simulink model "SWC_DID_type"  (R2021b)
settings: Solver=FixedStepDiscrete  StartTime=0.0  StopTime=10.0  RelTol=1e-3
(part 1 of 2)
settings Model: DataDictionary=APPTypes.sldd  Creator=FVT23033  LastModifiedBy=FVT23033
settings DataIOCC: SaveFormat=StructureWithTime
settings OptimizationCC: DefaultParameterBehavior=Inlined  EnhancedBackFolding=on  PassReuseOutputArgsAs=Individual arguments  ZeroExternalMemoryAtStartup=off  ZeroInternalMemoryAtStartup=off  OptimizeBlockOrder=speed  DifferentSizesBufferReuse=on  OptimizationCustomize=off  EfficientTunableParamExpr=on
settings DebuggingCC: ParameterTunabilityLossMsg=error
settings HardwareCC: ProdBitPerPointer=32  ProdBitPerSizeT=32  ProdBitPerPtrDiffT=32  ProdLargestAtomicInteger=Long  ProdLargestAtomicFloat=Double  ProdWordSize=32  ProdLongLongMode=on  ProdHWDeviceType=ARM Compatible->ARM Cortex-M
settings SFSimCC: MATLABDynamicMemAlloc=off
settings RTWCC: Description=AUTOSAR  SystemTargetFile=autosar.tlc  GenCodeOnly=on  TemplateMakefile=ert_default_tmf  PortableWordSizes=on
settings CodeAppCC: ForceParamTrailComments=on  IgnoreCustomStorageClasses=off  OperatorAnnotations=on  SimulinkDataObjDesc=on  SFDataObjDesc=on  InsertBlockDesc=on
settings STFCustomTargetCC: TargetLangStandard=C99 (ISO)  UtilityFuncGeneration=Shared location  MultiwordLength=256  ParMdlRefBuildCompliant=on  CompOptLevelCompliant=on  IncludeMdlTerminateFcn=off  CombineOutputUpdateFcns=on  SuppressErrorStatus=on  ERTCustomFileBanners=on  SupportNonFinite=off  SupportComplex=off  SupportContinuousTime=off  SupportNonInlinedSFcns=off  RemoveResetFunc=on  MATLABClassNameForMDSCustomization=Simulink.SoftwareTarget.ERTCustomization  AutosarCompliant=on  GRTInterface=off  UseToolchainInfoCompliant=on  GenerateSharedConstants=off  LookupTableObjectStructAxisOrder=2,1,3,4,...  LUTObjectStructOrderEvenSpacing=Size,Table,Breakpoints  SystemTargetFile=autosar.tlc
settings ERTTargetCC: TargetLangStandard=C99 (ISO)  UtilityFuncGeneration=Shared location  ConcurrentExecutionCompliant=off  IncludeMdlTerminateFcn=off  SuppressErrorStatus=on  SupportNonFinite=off  SupportComplex=off  ModelStepFunctionPrototypeControlCompliant=off  CPPClassGenCompliant=off  AutosarCompliant=on  GenerateSharedConstants=off  LookupTableObjectStructAxisOrder=2,1,3,4,...  LUTObjectStructOrderEvenSpacing=Size,Table,Breakpoints  GenerateASAP2=on  InlinedParameterPlacement=NonHierarchical  ERTCustomFileTemplate=example_file_process.tlc  ConvertIfToSwitch=off  SuppressUnreachableDefaultCases=off  BooleanTrueId=true_MatlabRTW  BooleanFalseId=false_MatlabRTW

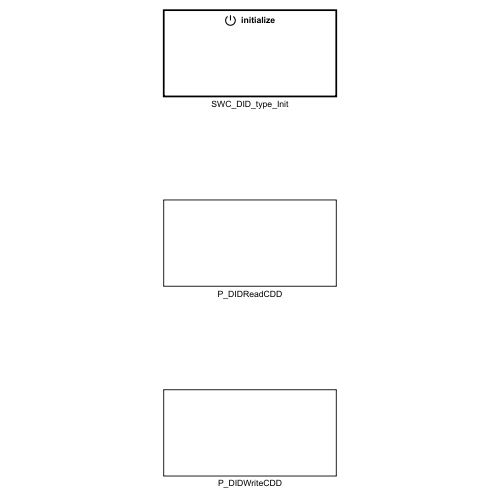
[thumbnail: Simulink's stored preview of the top-level diagram]
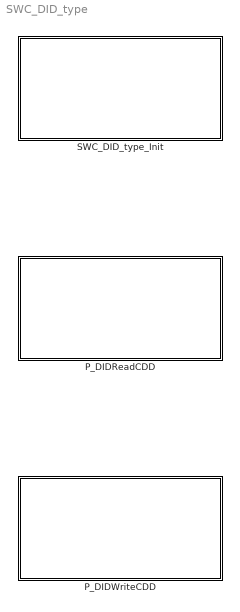
== system SWC_DID_type ==
  P_DIDReadCDD : Subsystem
  P_DIDWriteCDD : Subsystem
  SWC_DID_type_Init : Subsystem

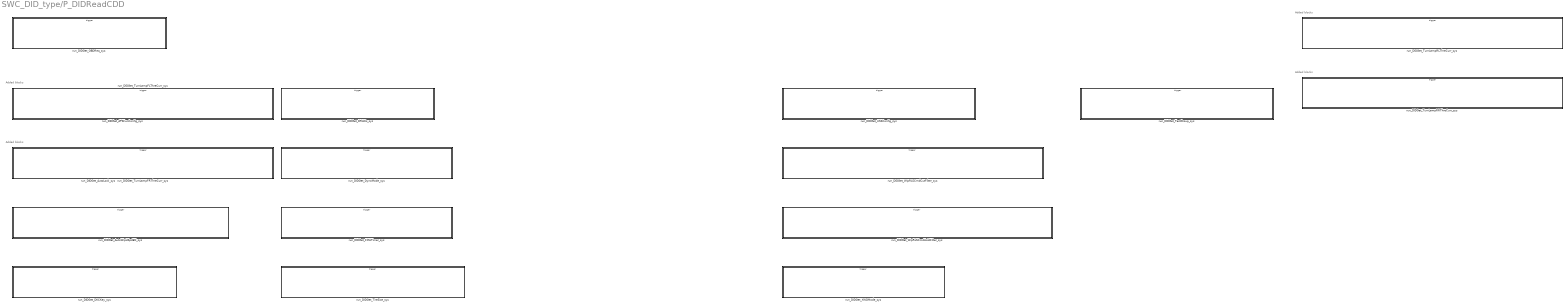
== system SWC_DID_type/P_DIDReadCDD ==
  note: Added blocks
  note: Added blocks
  note: Added blocks
  note: Added blocks
  run_DIDGet_APSFunConfig_sys : Subsystem
  run_DIDGet_AutoLock_sys : Subsystem
  run_DIDGet_AutoWipHSpdEN_sys : Subsystem
  run_DIDGet_DKCKey_sys : Subsystem
  run_DIDGet_DRLDis_sys : Subsystem
  run_DIDGet_DynoMode_sys : Subsystem
  run_DIDGet_FMHTimer_sys : Subsystem
  run_DIDGet_OBDReq_sys : Subsystem
  run_DIDGet_TestGroup_sys : Subsystem
  run_DIDGet_TireSize_sys : Subsystem
  run_DIDGet_TurnLampFLThreCurr_sys : Subsystem
  run_DIDGet_TurnLampFRThreCurr_sys : Subsystem
  run_DIDGet_TurnLampRLThreCurr_sys : Subsystem
  run_DIDGet_TurnLampRRThreCurr_sys : Subsystem
  run_DIDGet_USSConfig_sys : Subsystem
  run_DIDGet_WipRLSCmdCutFilter_sys : Subsystem
  run_DIDGet_WipRLSCmdHoldFilter_sys : Subsystem
  run_DIDGet_XWDMode_sys : Subsystem

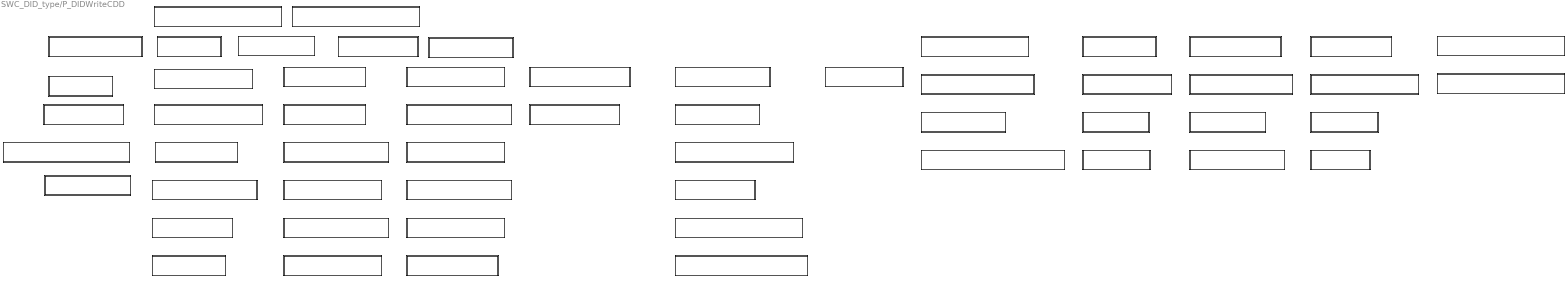
== system SWC_DID_type/P_DIDWriteCDD ==
  note: Added blocks
  note: Added blocks
  note: Added blocks
  note: Added blocks
  run_DIDSet_APPD_sys : Subsystem
  run_DIDSet_APPE_sys : Subsystem
  run_DIDSet_APPPedalZP_sys : Subsystem
  run_DIDSet_APSFunConfig_sys : Subsystem
  run_DIDSet_AutoLock_sys : Subsystem
  run_DIDSet_AutoWipHSpdEN_sys : Subsystem
  run_DIDSet_CALID_sys : Subsystem
  run_DIDSet_CDEODT_sys : Subsystem
  run_DIDSet_CLRDIST_sys : Subsystem
  run_DIDSet_DKCBLESta_sys : Subsystem
  run_DIDSet_DKCKey_sys : Subsystem
  run_DIDSet_DKCSta_sys : Subsystem
  run_DIDSet_DRLDis_sys : Subsystem
  run_DIDSet_DoorNFCAnchorSta_sys : Subsystem
  run_DIDSet_DynoMode_sys : Subsystem
  run_DIDSet_ECUNAME_sys : Subsystem
  run_DIDSet_FDDKCCoordXY_sys : Subsystem
  run_DIDSet_FMHTimer_sys : Subsystem
  run_DIDSet_LFLowPresThre_sys : Subsystem
  run_DIDSet_LFSensorID_sys : Subsystem
  run_DIDSet_LIDAAnchorSta_sys : Subsystem
  run_DIDSet_LRLowPresThre_sys : Subsystem
  run_DIDSet_LRSensorID_sys : Subsystem
  run_DIDSet_MILDIST_sys : Subsystem
  run_DIDSet_NUMPSATRIPSFLTMEMCLR_sys : Subsystem
  run_DIDSet_NVMPedalZP_sys : Subsystem
  run_DIDSet_OBDReq_sys : Subsystem
  run_DIDSet_ODOMETER_sys : Subsystem
  run_DIDSet_PKE_sys : Subsystem
  run_DIDSet_PSA_sys : Subsystem
  run_DIDSet_ProtocolId_sys : Subsystem
  run_DIDSet_QTYPSATRIPS_sys : Subsystem
  run_DIDSet_RFLowPresThre_sys : Subsystem
  run_DIDSet_RFSensorID_sys : Subsystem
  run_DIDSet_RRLowPresThre_sys : Subsystem
  run_DIDSet_RRSensorID_sys : Subsystem
  run_DIDSet_RUNTM_sys : Subsystem
  run_DIDSet_SensorMode_sys : Subsystem
  run_DIDSet_TPMSLearnSta_sys : Subsystem
  run_DIDSet_TestGroup_sys : Subsystem
  run_DIDSet_TireSize_sys : Subsystem
  run_DIDSet_TurnLampFLThreCurr_sys : Subsystem
  run_DIDSet_TurnLampFRThreCurr_sys : Subsystem
  run_DIDSet_TurnLampRLThreCurr_sys : Subsystem
  run_DIDSet_TurnLampRRThreCurr_sys : Subsystem
  run_DIDSet_UIDSta_sys : Subsystem
  run_DIDSet_USSConfig_sys : Subsystem
  run_DIDSet_UWBAnchorSta_sys : Subsystem
  run_DIDSet_VIN_sys : Subsystem
  run_DIDSet_VSS_sys : Subsystem
  run_DIDSet_WhlPres_sys : Subsystem
  run_DIDSet_WhlSensorBattSta_sys : Subsystem
  run_DIDSet_WhlTmp_sys : Subsystem
  run_DIDSet_WipRLSCmdCutFilter_sys : Subsystem
  run_DIDSet_WipRLSCmdHoldFilter_sys : Subsystem
  run_DIDSet_XWDMode_sys : Subsystem

== system SWC_DID_type/SWC_DID_type_Init ==
  Event Listener : EventListener  EventName=reset

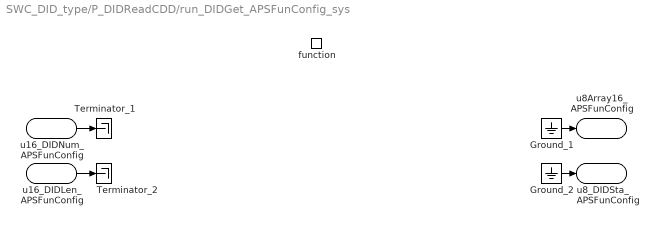
== system SWC_DID_type/P_DIDReadCDD/run_DIDGet_APSFunConfig_sys ==
  function : TriggerPort  TriggerType=function-call  IsSimulinkFunction=on  FunctionName=run_DIDGet_APSFunConfig  VariantControl=(inherit)
  Ground_1 : Ground
  Ground_2 : Ground
  Terminator_1 : Terminator
  Terminator_2 : Terminator
  u16_DIDNum_APSFunConfig : ArgIn  OutDataTypeStr=uint16  ArgumentName=u16_DIDNum_APSFunConfig
  u16_DIDLen_APSFunConfig : ArgIn  Port=2  OutDataTypeStr=uint16  ArgumentName=u16_DIDLen_APSFunConfig
  u8Array16_APSFunConfig : ArgOut  OutDataTypeStr=uint8  PortDimensions=16  ArgumentName=u8Array16_APSFunConfig
  u8_DIDSta_APSFunConfig : ArgOut  Port=2  OutDataTypeStr=uint8  ArgumentName=u8_DIDSta_APSFunConfig
  wires:
  u16_DIDNum_APSFunConfig/1 -> Terminator_1/1
  u16_DIDLen_APSFunConfig/1 -> Terminator_2/1
  Ground_1/1 -> u8Array16_APSFunConfig/1
  Ground_2/1 -> u8_DIDSta_APSFunConfig/1

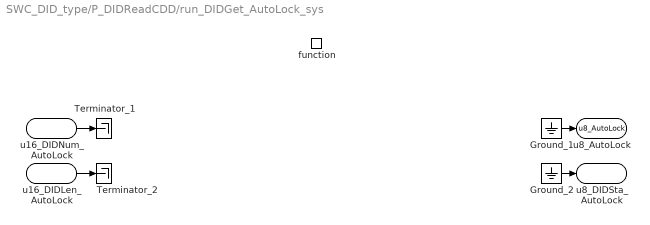
== system SWC_DID_type/P_DIDReadCDD/run_DIDGet_AutoLock_sys ==
  function : TriggerPort  TriggerType=function-call  IsSimulinkFunction=on  FunctionName=run_DIDGet_AutoLock  VariantControl=(inherit)
  Ground_1 : Ground
  Ground_2 : Ground
  Terminator_1 : Terminator
  Terminator_2 : Terminator
  u16_DIDNum_AutoLock : ArgIn  OutDataTypeStr=uint16  ArgumentName=u16_DIDNum_AutoLock
  u16_DIDLen_AutoLock : ArgIn  Port=2  OutDataTypeStr=uint16  ArgumentName=u16_DIDLen_AutoLock
  u8_AutoLock : ArgOut  OutDataTypeStr=uint8  ArgumentName=u8_AutoLock
  u8_DIDSta_AutoLock : ArgOut  Port=2  OutDataTypeStr=uint8  ArgumentName=u8_DIDSta_AutoLock
  wires:
  u16_DIDNum_AutoLock/1 -> Terminator_1/1
  u16_DIDLen_AutoLock/1 -> Terminator_2/1
  Ground_1/1 -> u8_AutoLock/1
  Ground_2/1 -> u8_DIDSta_AutoLock/1

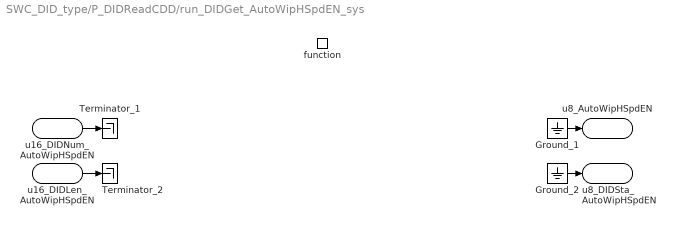
== system SWC_DID_type/P_DIDReadCDD/run_DIDGet_AutoWipHSpdEN_sys ==
  function : TriggerPort  TriggerType=function-call  IsSimulinkFunction=on  FunctionName=run_DIDGet_AutoWipHSpdEN  VariantControl=(inherit)
  Ground_1 : Ground
  Ground_2 : Ground
  Terminator_1 : Terminator
  Terminator_2 : Terminator
  u16_DIDNum_AutoWipHSpdEN : ArgIn  OutDataTypeStr=uint16  ArgumentName=u16_DIDNum_AutoWipHSpdEN
  u16_DIDLen_AutoWipHSpdEN : ArgIn  Port=2  OutDataTypeStr=uint16  ArgumentName=u16_DIDLen_AutoWipHSpdEN
  u8_AutoWipHSpdEN : ArgOut  OutDataTypeStr=uint8  ArgumentName=u8_AutoWipHSpdEN
  u8_DIDSta_AutoWipHSpdEN : ArgOut  Port=2  OutDataTypeStr=uint8  ArgumentName=u8_DIDSta_AutoWipHSpdEN
  wires:
  u16_DIDNum_AutoWipHSpdEN/1 -> Terminator_1/1
  u16_DIDLen_AutoWipHSpdEN/1 -> Terminator_2/1
  Ground_1/1 -> u8_AutoWipHSpdEN/1
  Ground_2/1 -> u8_DIDSta_AutoWipHSpdEN/1

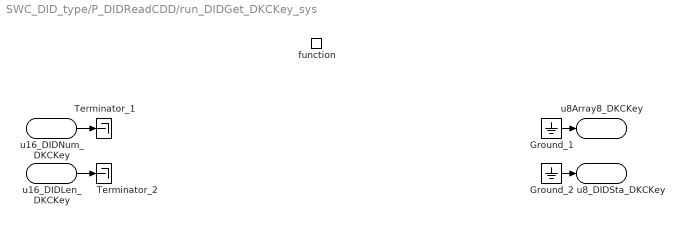
== system SWC_DID_type/P_DIDReadCDD/run_DIDGet_DKCKey_sys ==
  function : TriggerPort  TriggerType=function-call  IsSimulinkFunction=on  FunctionName=run_DIDGet_DKCKey  VariantControl=(inherit)
  Ground_1 : Ground
  Ground_2 : Ground
  Terminator_1 : Terminator
  Terminator_2 : Terminator
  u16_DIDNum_DKCKey : ArgIn  OutDataTypeStr=uint16  ArgumentName=u16_DIDNum_DKCKey
  u16_DIDLen_DKCKey : ArgIn  Port=2  OutDataTypeStr=uint16  ArgumentName=u16_DIDLen_DKCKey
  u8Array8_DKCKey : ArgOut  OutDataTypeStr=uint8  PortDimensions=8  ArgumentName=u8Array8_DKCKey
  u8_DIDSta_DKCKey : ArgOut  Port=2  OutDataTypeStr=uint8  ArgumentName=u8_DIDSta_DKCKey
  wires:
  u16_DIDNum_DKCKey/1 -> Terminator_1/1
  u16_DIDLen_DKCKey/1 -> Terminator_2/1
  Ground_1/1 -> u8Array8_DKCKey/1
  Ground_2/1 -> u8_DIDSta_DKCKey/1

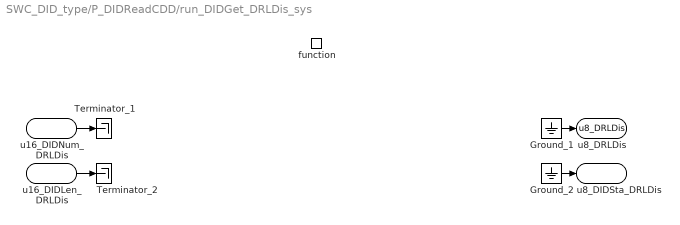
== system SWC_DID_type/P_DIDReadCDD/run_DIDGet_DRLDis_sys ==
  function : TriggerPort  TriggerType=function-call  IsSimulinkFunction=on  FunctionName=run_DIDGet_DRLDis  VariantControl=(inherit)
  Ground_1 : Ground
  Ground_2 : Ground
  Terminator_1 : Terminator
  Terminator_2 : Terminator
  u16_DIDNum_DRLDis : ArgIn  OutDataTypeStr=uint16  ArgumentName=u16_DIDNum_DRLDis
  u16_DIDLen_DRLDis : ArgIn  Port=2  OutDataTypeStr=uint16  ArgumentName=u16_DIDLen_DRLDis
  u8_DRLDis : ArgOut  OutDataTypeStr=uint8  ArgumentName=u8_DRLDis
  u8_DIDSta_DRLDis : ArgOut  Port=2  OutDataTypeStr=uint8  ArgumentName=u8_DIDSta_DRLDis
  wires:
  u16_DIDNum_DRLDis/1 -> Terminator_1/1
  u16_DIDLen_DRLDis/1 -> Terminator_2/1
  Ground_1/1 -> u8_DRLDis/1
  Ground_2/1 -> u8_DIDSta_DRLDis/1

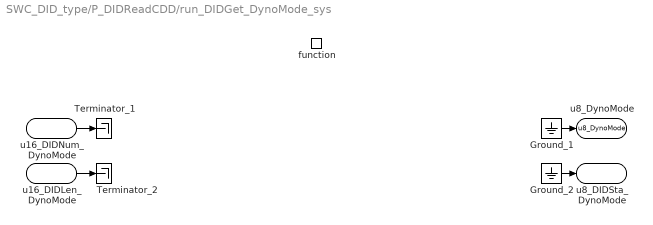
== system SWC_DID_type/P_DIDReadCDD/run_DIDGet_DynoMode_sys ==
  function : TriggerPort  TriggerType=function-call  IsSimulinkFunction=on  FunctionName=run_DIDGet_DynoMode  VariantControl=(inherit)
  Ground_1 : Ground
  Ground_2 : Ground
  Terminator_1 : Terminator
  Terminator_2 : Terminator
  u16_DIDNum_DynoMode : ArgIn  OutDataTypeStr=uint16  ArgumentName=u16_DIDNum_DynoMode
  u16_DIDLen_DynoMode : ArgIn  Port=2  OutDataTypeStr=uint16  ArgumentName=u16_DIDLen_DynoMode
  u8_DynoMode : ArgOut  OutDataTypeStr=uint8  ArgumentName=u8_DynoMode
  u8_DIDSta_DynoMode : ArgOut  Port=2  OutDataTypeStr=uint8  ArgumentName=u8_DIDSta_DynoMode
  wires:
  u16_DIDNum_DynoMode/1 -> Terminator_1/1
  u16_DIDLen_DynoMode/1 -> Terminator_2/1
  Ground_1/1 -> u8_DynoMode/1
  Ground_2/1 -> u8_DIDSta_DynoMode/1

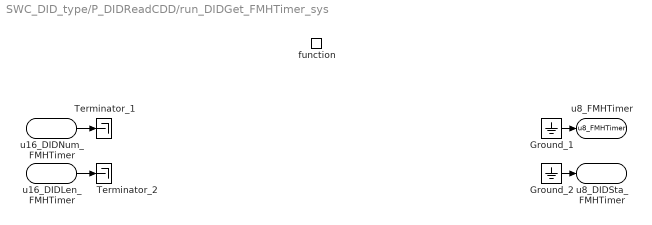
== system SWC_DID_type/P_DIDReadCDD/run_DIDGet_FMHTimer_sys ==
  function : TriggerPort  TriggerType=function-call  IsSimulinkFunction=on  FunctionName=run_DIDGet_FMHTimer  VariantControl=(inherit)
  Ground_1 : Ground
  Ground_2 : Ground
  Terminator_1 : Terminator
  Terminator_2 : Terminator
  u16_DIDNum_FMHTimer : ArgIn  OutDataTypeStr=uint16  ArgumentName=u16_DIDNum_FMHTimer
  u16_DIDLen_FMHTimer : ArgIn  Port=2  OutDataTypeStr=uint16  ArgumentName=u16_DIDLen_FMHTimer
  u8_FMHTimer : ArgOut  OutDataTypeStr=uint8  ArgumentName=u8_FMHTimer
  u8_DIDSta_FMHTimer : ArgOut  Port=2  OutDataTypeStr=uint8  ArgumentName=u8_DIDSta_FMHTimer
  wires:
  u16_DIDNum_FMHTimer/1 -> Terminator_1/1
  u16_DIDLen_FMHTimer/1 -> Terminator_2/1
  Ground_1/1 -> u8_FMHTimer/1
  Ground_2/1 -> u8_DIDSta_FMHTimer/1

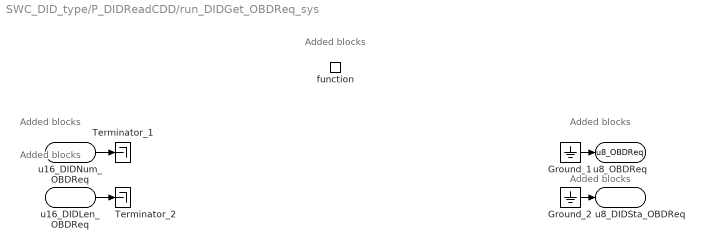
== system SWC_DID_type/P_DIDReadCDD/run_DIDGet_OBDReq_sys ==
  note: Added blocks
  note: Added blocks
  note: Added blocks
  note: Added blocks
  note: Added blocks
  function : TriggerPort  TriggerType=function-call  IsSimulinkFunction=on  FunctionName=run_DIDGet_OBDReq  VariantControl=(inherit)
  Ground_1 : Ground
  Ground_2 : Ground
  Terminator_1 : Terminator
  Terminator_2 : Terminator
  u16_DIDNum_OBDReq : ArgIn  OutDataTypeStr=uint16  ArgumentName=u16_DIDNum_OBDReq
  u16_DIDLen_OBDReq : ArgIn  Port=2  OutDataTypeStr=uint16  ArgumentName=u16_DIDLen_OBDReq
  u8_OBDReq : ArgOut  OutDataTypeStr=uint8  ArgumentName=u8_OBDReq
  u8_DIDSta_OBDReq : ArgOut  Port=2  OutDataTypeStr=uint8  ArgumentName=u8_DIDSta_OBDReq
  wires:
  u16_DIDNum_OBDReq/1 -> Terminator_1/1
  u16_DIDLen_OBDReq/1 -> Terminator_2/1
  Ground_1/1 -> u8_OBDReq/1
  Ground_2/1 -> u8_DIDSta_OBDReq/1

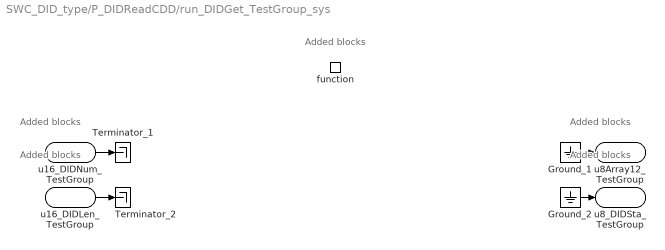
== system SWC_DID_type/P_DIDReadCDD/run_DIDGet_TestGroup_sys ==
  note: Added blocks
  note: Added blocks
  note: Added blocks
  note: Added blocks
  note: Added blocks
  function : TriggerPort  TriggerType=function-call  IsSimulinkFunction=on  FunctionName=run_DIDGet_TestGroup  VariantControl=(inherit)
  Ground_1 : Ground
  Ground_2 : Ground
  Terminator_1 : Terminator
  Terminator_2 : Terminator
  u16_DIDNum_TestGroup : ArgIn  OutDataTypeStr=uint16  ArgumentName=u16_DIDNum_TestGroup
  u16_DIDLen_TestGroup : ArgIn  Port=2  OutDataTypeStr=uint16  ArgumentName=u16_DIDLen_TestGroup
  u8Array12_TestGroup : ArgOut  OutDataTypeStr=uint8  PortDimensions=12  ArgumentName=u8Array12_TestGroup
  u8_DIDSta_TestGroup : ArgOut  Port=2  OutDataTypeStr=uint8  ArgumentName=u8_DIDSta_TestGroup
  wires:
  u16_DIDNum_TestGroup/1 -> Terminator_1/1
  u16_DIDLen_TestGroup/1 -> Terminator_2/1
  Ground_1/1 -> u8Array12_TestGroup/1
  Ground_2/1 -> u8_DIDSta_TestGroup/1

== system SWC_DID_type/P_DIDReadCDD/run_DIDGet_TireSize_sys ==
  function : TriggerPort  TriggerType=function-call  IsSimulinkFunction=on  FunctionName=run_DIDGet_TireSize  VariantControl=(inherit)
  Ground_1 : Ground
  Ground_2 : Ground
  Terminator_1 : Terminator
  Terminator_2 : Terminator
  u16_DIDNum_TireSize : ArgIn  OutDataTypeStr=uint16  ArgumentName=u16_DIDNum_TireSize
  u16_DIDLen_TireSize : ArgIn  Port=2  OutDataTypeStr=uint16  ArgumentName=u16_DIDLen_TireSize
  u8Array16_TireSize : ArgOut  OutDataTypeStr=uint8  PortDimensions=16  ArgumentName=u8Array16_TireSize
  u8_DIDSta_TireSize : ArgOut  Port=2  OutDataTypeStr=uint8  ArgumentName=u8_DIDSta_TireSize
  wires:
  u16_DIDNum_TireSize/1 -> Terminator_1/1
  u16_DIDLen_TireSize/1 -> Terminator_2/1
  Ground_1/1 -> u8Array16_TireSize/1
  Ground_2/1 -> u8_DIDSta_TireSize/1

== system SWC_DID_type/P_DIDReadCDD/run_DIDGet_TurnLampFLThreCurr_sys ==
  note: Added blocks
  note: Added blocks
  note: Added blocks
  note: Added blocks
  note: Added blocks
  function : TriggerPort  TriggerType=function-call  IsSimulinkFunction=on  FunctionName=run_DIDGet_TurnLampFLThreCurr  VariantControl=(inherit)
  Ground_1 : Ground
  Ground_2 : Ground
  Terminator_1 : Terminator
  Terminator_2 : Terminator
  u16_DIDNum_TurnLampFLThreCurr : ArgIn  OutDataTypeStr=uint16  ArgumentName=u16_DIDNum_TurnLampFLThreCurr
  u16_DIDLen_TurnLampFLThreCurr : ArgIn  Port=2  OutDataTypeStr=uint16  ArgumentName=u16_DIDLen_TurnLampFLThreCurr
  u8_TurnLampFLThreCurr : ArgOut  OutDataTypeStr=uint8  ArgumentName=u8_TurnLampFLThreCurr
  u8_DIDSta_TurnLampFLThreCurr : ArgOut  Port=2  OutDataTypeStr=uint8  ArgumentName=u8_DIDSta_TurnLampFLThreCurr
  wires:
  u16_DIDNum_TurnLampFLThreCurr/1 -> Terminator_1/1
  u16_DIDLen_TurnLampFLThreCurr/1 -> Terminator_2/1
  Ground_1/1 -> u8_TurnLampFLThreCurr/1
  Ground_2/1 -> u8_DIDSta_TurnLampFLThreCurr/1

== system SWC_DID_type/P_DIDReadCDD/run_DIDGet_TurnLampFRThreCurr_sys ==
  note: Added blocks
  note: Added blocks
  note: Added blocks
  note: Added blocks
  note: Added blocks
  function : TriggerPort  TriggerType=function-call  IsSimulinkFunction=on  FunctionName=run_DIDGet_TurnLampFRThreCurr  VariantControl=(inherit)
  Ground_1 : Ground
  Ground_2 : Ground
  Terminator_1 : Terminator
  Terminator_2 : Terminator
  u16_DIDNum_TurnLampFRThreCurr : ArgIn  OutDataTypeStr=uint16  ArgumentName=u16_DIDNum_TurnLampFRThreCurr
  u16_DIDLen_TurnLampFRThreCurr : ArgIn  Port=2  OutDataTypeStr=uint16  ArgumentName=u16_DIDLen_TurnLampFRThreCurr
  u8_TurnLampFRThreCurr : ArgOut  OutDataTypeStr=uint8  ArgumentName=u8_TurnLampFRThreCurr
  u8_DIDSta_TurnLampFRThreCurr : ArgOut  Port=2  OutDataTypeStr=uint8  ArgumentName=u8_DIDSta_TurnLampFRThreCurr
  wires:
  u16_DIDNum_TurnLampFRThreCurr/1 -> Terminator_1/1
  u16_DIDLen_TurnLampFRThreCurr/1 -> Terminator_2/1
  Ground_1/1 -> u8_TurnLampFRThreCurr/1
  Ground_2/1 -> u8_DIDSta_TurnLampFRThreCurr/1

== system SWC_DID_type/P_DIDReadCDD/run_DIDGet_TurnLampRLThreCurr_sys ==
  note: Added blocks
  note: Added blocks
  note: Added blocks
  note: Added blocks
  note: Added blocks
  function : TriggerPort  TriggerType=function-call  IsSimulinkFunction=on  FunctionName=run_DIDGet_TurnLampRLThreCurr  VariantControl=(inherit)
  Ground_1 : Ground
  Ground_2 : Ground
  Terminator_1 : Terminator
  Terminator_2 : Terminator
  u16_DIDNum_TurnLampRLThreCurr : ArgIn  OutDataTypeStr=uint16  ArgumentName=u16_DIDNum_TurnLampRLThreCurr
  u16_DIDLen_TurnLampRLThreCurr : ArgIn  Port=2  OutDataTypeStr=uint16  ArgumentName=u16_DIDLen_TurnLampRLThreCurr
  u8_TurnLampRLThreCurr : ArgOut  OutDataTypeStr=uint8  ArgumentName=u8_TurnLampRLThreCurr
  u8_DIDSta_TurnLampRLThreCurr : ArgOut  Port=2  OutDataTypeStr=uint8  ArgumentName=u8_DIDSta_TurnLampRLThreCurr
  wires:
  u16_DIDNum_TurnLampRLThreCurr/1 -> Terminator_1/1
  u16_DIDLen_TurnLampRLThreCurr/1 -> Terminator_2/1
  Ground_1/1 -> u8_TurnLampRLThreCurr/1
  Ground_2/1 -> u8_DIDSta_TurnLampRLThreCurr/1

== system SWC_DID_type/P_DIDReadCDD/run_DIDGet_TurnLampRRThreCurr_sys ==
  note: Added blocks
  note: Added blocks
  note: Added blocks
  note: Added blocks
  note: Added blocks
  function : TriggerPort  TriggerType=function-call  IsSimulinkFunction=on  FunctionName=run_DIDGet_TurnLampRRThreCurr  VariantControl=(inherit)
  Ground_1 : Ground
  Ground_2 : Ground
  Terminator_1 : Terminator
  Terminator_2 : Terminator
  u16_DIDNum_TurnLampRRThreCurr : ArgIn  OutDataTypeStr=uint16  ArgumentName=u16_DIDNum_TurnLampRRThreCurr
  u16_DIDLen_TurnLampRRThreCurr : ArgIn  Port=2  OutDataTypeStr=uint16  ArgumentName=u16_DIDLen_TurnLampRRThreCurr
  u8_TurnLampRRThreCurr : ArgOut  OutDataTypeStr=uint8  ArgumentName=u8_TurnLampRRThreCurr
  u8_DIDSta_TurnLampRRThreCurr : ArgOut  Port=2  OutDataTypeStr=uint8  ArgumentName=u8_DIDSta_TurnLampRRThreCurr
  wires:
  u16_DIDNum_TurnLampRRThreCurr/1 -> Terminator_1/1
  u16_DIDLen_TurnLampRRThreCurr/1 -> Terminator_2/1
  Ground_1/1 -> u8_TurnLampRRThreCurr/1
  Ground_2/1 -> u8_DIDSta_TurnLampRRThreCurr/1

== system SWC_DID_type/P_DIDReadCDD/run_DIDGet_USSConfig_sys ==
  function : TriggerPort  TriggerType=function-call  IsSimulinkFunction=on  FunctionName=run_DIDGet_USSConfig  VariantControl=(inherit)
  Ground_1 : Ground
  Ground_2 : Ground
  Terminator_1 : Terminator
  Terminator_2 : Terminator
  u16_DIDNum_USSConfig : ArgIn  OutDataTypeStr=uint16  ArgumentName=u16_DIDNum_USSConfig
  u16_DIDLen_USSConfig : ArgIn  Port=2  OutDataTypeStr=uint16  ArgumentName=u16_DIDLen_USSConfig
  u8Array16_USSConfig : ArgOut  OutDataTypeStr=uint8  PortDimensions=16  ArgumentName=u8Array16_USSConfig
  u8_DIDSta_USSConfig : ArgOut  Port=2  OutDataTypeStr=uint8  ArgumentName=u8_DIDSta_USSConfig
  wires:
  u16_DIDNum_USSConfig/1 -> Terminator_1/1
  u16_DIDLen_USSConfig/1 -> Terminator_2/1
  Ground_1/1 -> u8Array16_USSConfig/1
  Ground_2/1 -> u8_DIDSta_USSConfig/1

== system SWC_DID_type/P_DIDReadCDD/run_DIDGet_WipRLSCmdCutFilter_sys ==
  function : TriggerPort  TriggerType=function-call  IsSimulinkFunction=on  FunctionName=run_DIDGet_WipRLSCmdCutFilter  VariantControl=(inherit)
  Ground_1 : Ground
  Ground_2 : Ground
  Terminator_1 : Terminator
  Terminator_2 : Terminator
  u16_DIDNum_WipRLSCmdCutFilter : ArgIn  OutDataTypeStr=uint16  ArgumentName=u16_DIDNum_WipRLSCmdCutFilter
  u16_DIDLen_WipRLSCmdCutFilter : ArgIn  Port=2  OutDataTypeStr=uint16  ArgumentName=u16_DIDLen_WipRLSCmdCutFilter
  u8_WipRLSCmdCutFilter : ArgOut  OutDataTypeStr=uint8  ArgumentName=u8_WipRLSCmdCutFilter
  u8_DIDSta_WipRLSCmdCutFilter : ArgOut  Port=2  OutDataTypeStr=uint8  ArgumentName=u8_DIDSta_WipRLSCmdCutFilter
  wires:
  u16_DIDNum_WipRLSCmdCutFilter/1 -> Terminator_1/1
  u16_DIDLen_WipRLSCmdCutFilter/1 -> Terminator_2/1
  Ground_1/1 -> u8_WipRLSCmdCutFilter/1
  Ground_2/1 -> u8_DIDSta_WipRLSCmdCutFilter/1

== system SWC_DID_type/P_DIDReadCDD/run_DIDGet_WipRLSCmdHoldFilter_sys ==
  function : TriggerPort  TriggerType=function-call  IsSimulinkFunction=on  FunctionName=run_DIDGet_WipRLSCmdHoldFilter  VariantControl=(inherit)
  Ground_1 : Ground
  Ground_2 : Ground
  Terminator_1 : Terminator
  Terminator_2 : Terminator
  u16_DIDNum_WipRLSCmdHoldFilter : ArgIn  OutDataTypeStr=uint16  ArgumentName=u16_DIDNum_WipRLSCmdHoldFilter
  u16_DIDLen_WipRLSCmdHoldFilter : ArgIn  Port=2  OutDataTypeStr=uint16  ArgumentName=u16_DIDLen_WipRLSCmdHoldFilter
  u8_WipRLSCmdHoldFilter : ArgOut  OutDataTypeStr=uint8  ArgumentName=u8_WipRLSCmdHoldFilter
  u8_DIDSta_WipRLSCmdHoldFilter : ArgOut  Port=2  OutDataTypeStr=uint8  ArgumentName=u8_DIDSta_WipRLSCmdHoldFilter
  wires:
  u16_DIDNum_WipRLSCmdHoldFilter/1 -> Terminator_1/1
  u16_DIDLen_WipRLSCmdHoldFilter/1 -> Terminator_2/1
  Ground_1/1 -> u8_WipRLSCmdHoldFilter/1
  Ground_2/1 -> u8_DIDSta_WipRLSCmdHoldFilter/1

== system SWC_DID_type/P_DIDReadCDD/run_DIDGet_XWDMode_sys ==
  function : TriggerPort  TriggerType=function-call  IsSimulinkFunction=on  FunctionName=run_DIDGet_XWDMode  VariantControl=(inherit)
  Ground_1 : Ground
  Ground_2 : Ground
  Terminator_1 : Terminator
  Terminator_2 : Terminator
  u16_DIDNum_XWDMode : ArgIn  OutDataTypeStr=uint16  ArgumentName=u16_DIDNum_XWDMode
  u16_DIDLen_XWDMode : ArgIn  Port=2  OutDataTypeStr=uint16  ArgumentName=u16_DIDLen_XWDMode
  u8_XWDMode : ArgOut  OutDataTypeStr=uint8  ArgumentName=u8_XWDMode
  u8_DIDSta_XWDMode : ArgOut  Port=2  OutDataTypeStr=uint8  ArgumentName=u8_DIDSta_XWDMode
  wires:
  u16_DIDNum_XWDMode/1 -> Terminator_1/1
  u16_DIDLen_XWDMode/1 -> Terminator_2/1
  Ground_1/1 -> u8_XWDMode/1
  Ground_2/1 -> u8_DIDSta_XWDMode/1

== system SWC_DID_type/P_DIDWriteCDD/run_DIDSet_APPD_sys ==
  note: Added blocks
  note: Added blocks
  note: Added blocks
  note: Added blocks
  function : TriggerPort  TriggerType=function-call  IsSimulinkFunction=on  FunctionName=run_DIDSet_APPD  VariantControl=(inherit)
  Terminator_1 : Terminator
  Terminator_2 : Terminator
  Terminator_3 : Terminator
  u16_DIDNum_APPD : ArgIn  OutDataTypeStr=uint16  ArgumentName=u16_DIDNum_APPD
  u16_DIDLen_APPD : ArgIn  Port=2  OutDataTypeStr=uint16  ArgumentName=u16_DIDLen_APPD
  u8_APPD : ArgIn  Port=3  OutDataTypeStr=uint8  ArgumentName=u8_APPD
  wires:
  u16_DIDNum_APPD/1 -> Terminator_1/1
  u16_DIDLen_APPD/1 -> Terminator_2/1
  u8_APPD/1 -> Terminator_3/1

== system SWC_DID_type/P_DIDWriteCDD/run_DIDSet_APPE_sys ==
  note: Added blocks
  note: Added blocks
  note: Added blocks
  note: Added blocks
  function : TriggerPort  TriggerType=function-call  IsSimulinkFunction=on  FunctionName=run_DIDSet_APPE  VariantControl=(inherit)
  Terminator_1 : Terminator
  Terminator_2 : Terminator
  Terminator_3 : Terminator
  u16_DIDNum_APPE : ArgIn  OutDataTypeStr=uint16  ArgumentName=u16_DIDNum_APPE
  u16_DIDLen_APPE : ArgIn  Port=2  OutDataTypeStr=uint16  ArgumentName=u16_DIDLen_APPE
  u8_APPE : ArgIn  Port=3  OutDataTypeStr=uint8  ArgumentName=u8_APPE
  wires:
  u16_DIDNum_APPE/1 -> Terminator_1/1
  u16_DIDLen_APPE/1 -> Terminator_2/1
  u8_APPE/1 -> Terminator_3/1

== system SWC_DID_type/P_DIDWriteCDD/run_DIDSet_APPPedalZP_sys ==
  function : TriggerPort  TriggerType=function-call  IsSimulinkFunction=on  FunctionName=run_DIDSet_APPPedalZP  VariantControl=(inherit)
  Terminator_1 : Terminator
  Terminator_2 : Terminator
  Terminator_3 : Terminator
  u16_DIDNum_APPPedalZP : ArgIn  OutDataTypeStr=uint16  ArgumentName=u16_DIDNum_APPPedalZP
  u16_DIDLen_APPPedalZP : ArgIn  Port=2  OutDataTypeStr=uint16  ArgumentName=u16_DIDLen_APPPedalZP
  u8Array3_APPPedalZP : ArgIn  Port=3  OutDataTypeStr=uint8  PortDimensions=3  ArgumentName=u8Array3_APPPedalZP
  wires:
  u16_DIDNum_APPPedalZP/1 -> Terminator_1/1
  u16_DIDLen_APPPedalZP/1 -> Terminator_2/1
  u8Array3_APPPedalZP/1 -> Terminator_3/1

== system SWC_DID_type/P_DIDWriteCDD/run_DIDSet_APSFunConfig_sys ==
  function : TriggerPort  TriggerType=function-call  IsSimulinkFunction=on  FunctionName=run_DIDSet_APSFunConfig  VariantControl=(inherit)
  Terminator_1 : Terminator
  Terminator_2 : Terminator
  Terminator_3 : Terminator
  u16_DIDNum_APSFunConfig : ArgIn  OutDataTypeStr=uint16  ArgumentName=u16_DIDNum_APSFunConfig
  u16_DIDLen_APSFunConfig : ArgIn  Port=2  OutDataTypeStr=uint16  ArgumentName=u16_DIDLen_APSFunConfig
  u8Array16_APSFunConfig : ArgIn  Port=3  OutDataTypeStr=uint8  PortDimensions=16  ArgumentName=u8Array16_APSFunConfig
  wires:
  u16_DIDNum_APSFunConfig/1 -> Terminator_1/1
  u16_DIDLen_APSFunConfig/1 -> Terminator_2/1
  u8Array16_APSFunConfig/1 -> Terminator_3/1

== system SWC_DID_type/P_DIDWriteCDD/run_DIDSet_AutoLock_sys ==
  function : TriggerPort  TriggerType=function-call  IsSimulinkFunction=on  FunctionName=run_DIDSet_AutoLock  VariantControl=(inherit)
  Terminator_1 : Terminator
  Terminator_2 : Terminator
  Terminator_3 : Terminator
  u16_DIDNum_AutoLock : ArgIn  OutDataTypeStr=uint16  ArgumentName=u16_DIDNum_AutoLock
  u16_DIDLen_AutoLock : ArgIn  Port=2  OutDataTypeStr=uint16  ArgumentName=u16_DIDLen_AutoLock
  u8_AutoLock : ArgIn  Port=3  OutDataTypeStr=uint8  ArgumentName=u8_AutoLock
  wires:
  u16_DIDNum_AutoLock/1 -> Terminator_1/1
  u16_DIDLen_AutoLock/1 -> Terminator_2/1
  u8_AutoLock/1 -> Terminator_3/1

== system SWC_DID_type/P_DIDWriteCDD/run_DIDSet_AutoWipHSpdEN_sys ==
  function : TriggerPort  TriggerType=function-call  IsSimulinkFunction=on  FunctionName=run_DIDSet_AutoWipHSpdEN  VariantControl=(inherit)
  Terminator_1 : Terminator
  Terminator_2 : Terminator
  Terminator_3 : Terminator
  u16_DIDNum_AutoWipHSpdEN : ArgIn  OutDataTypeStr=uint16  ArgumentName=u16_DIDNum_AutoWipHSpdEN
  u16_DIDLen_AutoWipHSpdEN : ArgIn  Port=2  OutDataTypeStr=uint16  ArgumentName=u16_DIDLen_AutoWipHSpdEN
  u8_AutoWipHSpdEN : ArgIn  Port=3  OutDataTypeStr=uint8  ArgumentName=u8_AutoWipHSpdEN
  wires:
  u16_DIDNum_AutoWipHSpdEN/1 -> Terminator_1/1
  u16_DIDLen_AutoWipHSpdEN/1 -> Terminator_2/1
  u8_AutoWipHSpdEN/1 -> Terminator_3/1

== system SWC_DID_type/P_DIDWriteCDD/run_DIDSet_CALID_sys ==
  note: Added blocks
  note: Added blocks
  note: Added blocks
  note: Added blocks
  function : TriggerPort  TriggerType=function-call  IsSimulinkFunction=on  FunctionName=run_DIDSet_CALID  VariantControl=(inherit)
  Terminator_1 : Terminator
  Terminator_2 : Terminator
  Terminator_3 : Terminator
  u16_DIDNum_CALID : ArgIn  OutDataTypeStr=uint16  ArgumentName=u16_DIDNum_CALID
  u16_DIDLen_CALID : ArgIn  Port=2  OutDataTypeStr=uint16  ArgumentName=u16_DIDLen_CALID
  u8Array16_CALID : ArgIn  Port=3  OutDataTypeStr=uint8  PortDimensions=16  ArgumentName=u8Array16_CALID
  wires:
  u16_DIDNum_CALID/1 -> Terminator_1/1
  u16_DIDLen_CALID/1 -> Terminator_2/1
  u8Array16_CALID/1 -> Terminator_3/1

== system SWC_DID_type/P_DIDWriteCDD/run_DIDSet_CDEODT_sys ==
  note: Added blocks
  note: Added blocks
  note: Added blocks
  note: Added blocks
  function : TriggerPort  TriggerType=function-call  IsSimulinkFunction=on  FunctionName=run_DIDSet_CDEODT  VariantControl=(inherit)
  Terminator_1 : Terminator
  Terminator_2 : Terminator
  Terminator_3 : Terminator
  u16_DIDNum_CDEODT : ArgIn  OutDataTypeStr=uint16  ArgumentName=u16_DIDNum_CDEODT
  u16_DIDLen_CDEODT : ArgIn  Port=2  OutDataTypeStr=uint16  ArgumentName=u16_DIDLen_CDEODT
  u8Array8_CDEODT : ArgIn  Port=3  OutDataTypeStr=uint8  PortDimensions=8  ArgumentName=u8Array8_CDEODT
  wires:
  u16_DIDNum_CDEODT/1 -> Terminator_1/1
  u16_DIDLen_CDEODT/1 -> Terminator_2/1
  u8Array8_CDEODT/1 -> Terminator_3/1

== system SWC_DID_type/P_DIDWriteCDD/run_DIDSet_CLRDIST_sys ==
  note: Added blocks
  note: Added blocks
  note: Added blocks
  note: Added blocks
  function : TriggerPort  TriggerType=function-call  IsSimulinkFunction=on  FunctionName=run_DIDSet_CLRDIST  VariantControl=(inherit)
  Terminator_1 : Terminator
  Terminator_2 : Terminator
  Terminator_3 : Terminator
  u16_DIDNum_CLRDIST : ArgIn  OutDataTypeStr=uint16  ArgumentName=u16_DIDNum_CLRDIST
  u16_DIDLen_CLRDIST : ArgIn  Port=2  OutDataTypeStr=uint16  ArgumentName=u16_DIDLen_CLRDIST
  u8Array2_CLRDIST : ArgIn  Port=3  OutDataTypeStr=uint8  PortDimensions=2  ArgumentName=u8Array2_CLRDIST
  wires:
  u16_DIDNum_CLRDIST/1 -> Terminator_1/1
  u16_DIDLen_CLRDIST/1 -> Terminator_2/1
  u8Array2_CLRDIST/1 -> Terminator_3/1

== system SWC_DID_type/P_DIDWriteCDD/run_DIDSet_DKCBLESta_sys ==
  note: Added blocks
  note: Added blocks
  note: Added blocks
  note: Added blocks
  function : TriggerPort  TriggerType=function-call  IsSimulinkFunction=on  FunctionName=run_DIDSet_DKCBLESta  VariantControl=(inherit)
  Terminator_1 : Terminator
  Terminator_2 : Terminator
  Terminator_3 : Terminator
  u16_DIDNum_DKCBLESta : ArgIn  OutDataTypeStr=uint16  ArgumentName=u16_DIDNum_DKCBLESta
  u16_DIDLen_DKCBLESta : ArgIn  Port=2  OutDataTypeStr=uint16  ArgumentName=u16_DIDLen_DKCBLESta
  u8Array2_DKCBLESta : ArgIn  Port=3  OutDataTypeStr=uint8  PortDimensions=2  ArgumentName=u8Array2_DKCBLESta
  wires:
  u16_DIDNum_DKCBLESta/1 -> Terminator_1/1
  u16_DIDLen_DKCBLESta/1 -> Terminator_2/1
  u8Array2_DKCBLESta/1 -> Terminator_3/1

== system SWC_DID_type/P_DIDWriteCDD/run_DIDSet_DKCKey_sys ==
  function : TriggerPort  TriggerType=function-call  IsSimulinkFunction=on  FunctionName=run_DIDSet_DKCKey  VariantControl=(inherit)
  Terminator_1 : Terminator
  Terminator_2 : Terminator
  Terminator_3 : Terminator
  u16_DIDNum_DKCKey : ArgIn  OutDataTypeStr=uint16  ArgumentName=u16_DIDNum_DKCKey
  u16_DIDLen_DKCKey : ArgIn  Port=2  OutDataTypeStr=uint16  ArgumentName=u16_DIDLen_DKCKey
  u8Array8_DKCKey : ArgIn  Port=3  OutDataTypeStr=uint8  PortDimensions=8  ArgumentName=u8Array8_DKCKey
  wires:
  u16_DIDNum_DKCKey/1 -> Terminator_1/1
  u16_DIDLen_DKCKey/1 -> Terminator_2/1
  u8Array8_DKCKey/1 -> Terminator_3/1

== system SWC_DID_type/P_DIDWriteCDD/run_DIDSet_DKCSta_sys ==
  note: Added blocks
  note: Added blocks
  note: Added blocks
  note: Added blocks
  function : TriggerPort  TriggerType=function-call  IsSimulinkFunction=on  FunctionName=run_DIDSet_DKCSta  VariantControl=(inherit)
  Terminator_1 : Terminator
  Terminator_2 : Terminator
  Terminator_3 : Terminator
  u16_DIDNum_DKCSta : ArgIn  OutDataTypeStr=uint16  ArgumentName=u16_DIDNum_DKCSta
  u16_DIDLen_DKCSta : ArgIn  Port=2  OutDataTypeStr=uint16  ArgumentName=u16_DIDLen_DKCSta
  u8Array2_DKCSta : ArgIn  Port=3  OutDataTypeStr=uint8  PortDimensions=2  ArgumentName=u8Array2_DKCSta
  wires:
  u16_DIDNum_DKCSta/1 -> Terminator_1/1
  u16_DIDLen_DKCSta/1 -> Terminator_2/1
  u8Array2_DKCSta/1 -> Terminator_3/1

== system SWC_DID_type/P_DIDWriteCDD/run_DIDSet_DRLDis_sys ==
  function : TriggerPort  TriggerType=function-call  IsSimulinkFunction=on  FunctionName=run_DIDSet_DRLDis  VariantControl=(inherit)
  Terminator_1 : Terminator
  Terminator_2 : Terminator
  Terminator_3 : Terminator
  u16_DIDNum_DRLDis : ArgIn  OutDataTypeStr=uint16  ArgumentName=u16_DIDNum_DRLDis
  u16_DIDLen_DRLDis : ArgIn  Port=2  OutDataTypeStr=uint16  ArgumentName=u16_DIDLen_DRLDis
  u8_DRLDis : ArgIn  Port=3  OutDataTypeStr=uint8  ArgumentName=u8_DRLDis
  wires:
  u16_DIDNum_DRLDis/1 -> Terminator_1/1
  u16_DIDLen_DRLDis/1 -> Terminator_2/1
  u8_DRLDis/1 -> Terminator_3/1

== system SWC_DID_type/P_DIDWriteCDD/run_DIDSet_DoorNFCAnchorSta_sys ==
  note: Added blocks
  note: Added blocks
  note: Added blocks
  note: Added blocks
  function : TriggerPort  TriggerType=function-call  IsSimulinkFunction=on  FunctionName=run_DIDSet_DoorNFCAnchorSta  VariantControl=(inherit)
  Terminator_1 : Terminator
  Terminator_2 : Terminator
  Terminator_3 : Terminator
  u16_DIDNum_DoorNFCAnchorSta : ArgIn  OutDataTypeStr=uint16  ArgumentName=u16_DIDNum_DoorNFCAnchorSta
  u16_DIDLen_DoorNFCAnchorSta : ArgIn  Port=2  OutDataTypeStr=uint16  ArgumentName=u16_DIDLen_DoorNFCAnchorSta
  u8Array21_DoorNFCAnchorSta : ArgIn  Port=3  OutDataTypeStr=uint8  PortDimensions=21  ArgumentName=u8Array21_DoorNFCAnchorSta
  wires:
  u16_DIDNum_DoorNFCAnchorSta/1 -> Terminator_1/1
  u16_DIDLen_DoorNFCAnchorSta/1 -> Terminator_2/1
  u8Array21_DoorNFCAnchorSta/1 -> Terminator_3/1

== system SWC_DID_type/P_DIDWriteCDD/run_DIDSet_DynoMode_sys ==
  function : TriggerPort  TriggerType=function-call  IsSimulinkFunction=on  FunctionName=run_DIDSet_DynoMode  VariantControl=(inherit)
  Terminator_1 : Terminator
  Terminator_2 : Terminator
  Terminator_3 : Terminator
  u16_DIDNum_DynoMode : ArgIn  OutDataTypeStr=uint16  ArgumentName=u16_DIDNum_DynoMode
  u16_DIDLen_DynoMode : ArgIn  Port=2  OutDataTypeStr=uint16  ArgumentName=u16_DIDLen_DynoMode
  u8_DynoMode : ArgIn  Port=3  OutDataTypeStr=uint8  ArgumentName=u8_DynoMode
  wires:
  u16_DIDNum_DynoMode/1 -> Terminator_1/1
  u16_DIDLen_DynoMode/1 -> Terminator_2/1
  u8_DynoMode/1 -> Terminator_3/1

== system SWC_DID_type/P_DIDWriteCDD/run_DIDSet_ECUNAME_sys ==
  note: Added blocks
  note: Added blocks
  note: Added blocks
  note: Added blocks
  function : TriggerPort  TriggerType=function-call  IsSimulinkFunction=on  FunctionName=run_DIDSet_ECUNAME  VariantControl=(inherit)
  Terminator_1 : Terminator
  Terminator_2 : Terminator
  Terminator_3 : Terminator
  u16_DIDNum_ECUNAME : ArgIn  OutDataTypeStr=uint16  ArgumentName=u16_DIDNum_ECUNAME
  u16_DIDLen_ECUNAME : ArgIn  Port=2  OutDataTypeStr=uint16  ArgumentName=u16_DIDLen_ECUNAME
  u8Array20_ECUNAME : ArgIn  Port=3  OutDataTypeStr=uint8  PortDimensions=20  ArgumentName=u8Array20_ECUNAME
  wires:
  u16_DIDNum_ECUNAME/1 -> Terminator_1/1
  u16_DIDLen_ECUNAME/1 -> Terminator_2/1
  u8Array20_ECUNAME/1 -> Terminator_3/1

== system SWC_DID_type/P_DIDWriteCDD/run_DIDSet_FDDKCCoordXY_sys ==
  note: Added blocks
  note: Added blocks
  note: Added blocks
  note: Added blocks
  function : TriggerPort  TriggerType=function-call  IsSimulinkFunction=on  FunctionName=run_DIDSet_FDDKCCoordXY  VariantControl=(inherit)
  Terminator_1 : Terminator
  Terminator_2 : Terminator
  Terminator_3 : Terminator
  u16_DIDNum_FDDKCCoordXY : ArgIn  OutDataTypeStr=uint16  ArgumentName=u16_DIDNum_FDDKCCoordXY
  u16_DIDLen_FDDKCCoordXY : ArgIn  Port=2  OutDataTypeStr=uint16  ArgumentName=u16_DIDLen_FDDKCCoordXY
  u8Array3_FDDKCCoordXY : ArgIn  Port=3  OutDataTypeStr=uint8  PortDimensions=3  ArgumentName=u8Array3_FDDKCCoordXY
  wires:
  u16_DIDNum_FDDKCCoordXY/1 -> Terminator_1/1
  u16_DIDLen_FDDKCCoordXY/1 -> Terminator_2/1
  u8Array3_FDDKCCoordXY/1 -> Terminator_3/1

== system SWC_DID_type/P_DIDWriteCDD/run_DIDSet_FMHTimer_sys ==
  function : TriggerPort  TriggerType=function-call  IsSimulinkFunction=on  FunctionName=run_DIDSet_FMHTimer  VariantControl=(inherit)
  Terminator_1 : Terminator
  Terminator_2 : Terminator
  Terminator_3 : Terminator
  u16_DIDNum_FMHTimer : ArgIn  OutDataTypeStr=uint16  ArgumentName=u16_DIDNum_FMHTimer
  u16_DIDLen_FMHTimer : ArgIn  Port=2  OutDataTypeStr=uint16  ArgumentName=u16_DIDLen_FMHTimer
  u8_FMHTimer : ArgIn  Port=3  OutDataTypeStr=uint8  ArgumentName=u8_FMHTimer
  wires:
  u16_DIDNum_FMHTimer/1 -> Terminator_1/1
  u16_DIDLen_FMHTimer/1 -> Terminator_2/1
  u8_FMHTimer/1 -> Terminator_3/1

== system SWC_DID_type/P_DIDWriteCDD/run_DIDSet_LFLowPresThre_sys ==
  function : TriggerPort  TriggerType=function-call  IsSimulinkFunction=on  FunctionName=run_DIDSet_LFLowPresThre  VariantControl=(inherit)
  Terminator_1 : Terminator
  Terminator_2 : Terminator
  Terminator_3 : Terminator
  u16_DIDNum_LFLowPresThre : ArgIn  OutDataTypeStr=uint16  ArgumentName=u16_DIDNum_LFLowPresThre
  u16_DIDLen_LFLowPresThre : ArgIn  Port=2  OutDataTypeStr=uint16  ArgumentName=u16_DIDLen_LFLowPresThre
  u8_LFLowPresThre : ArgIn  Port=3  OutDataTypeStr=uint8  ArgumentName=u8_LFLowPresThre
  wires:
  u16_DIDNum_LFLowPresThre/1 -> Terminator_1/1
  u16_DIDLen_LFLowPresThre/1 -> Terminator_2/1
  u8_LFLowPresThre/1 -> Terminator_3/1

== system SWC_DID_type/P_DIDWriteCDD/run_DIDSet_LFSensorID_sys ==
  function : TriggerPort  TriggerType=function-call  IsSimulinkFunction=on  FunctionName=run_DIDSet_LFSensorID  VariantControl=(inherit)
  Terminator_1 : Terminator
  Terminator_2 : Terminator
  Terminator_3 : Terminator
  u16_DIDNum_LFSensorID : ArgIn  OutDataTypeStr=uint16  ArgumentName=u16_DIDNum_LFSensorID
  u16_DIDLen_LFSensorID : ArgIn  Port=2  OutDataTypeStr=uint16  ArgumentName=u16_DIDLen_LFSensorID
  u8Array4_LFSensorID : ArgIn  Port=3  OutDataTypeStr=uint8  PortDimensions=4  ArgumentName=u8Array4_LFSensorID
  wires:
  u16_DIDNum_LFSensorID/1 -> Terminator_1/1
  u16_DIDLen_LFSensorID/1 -> Terminator_2/1
  u8Array4_LFSensorID/1 -> Terminator_3/1

== system SWC_DID_type/P_DIDWriteCDD/run_DIDSet_LIDAAnchorSta_sys ==
  note: Added blocks
  note: Added blocks
  note: Added blocks
  note: Added blocks
  function : TriggerPort  TriggerType=function-call  IsSimulinkFunction=on  FunctionName=run_DIDSet_LIDAAnchorSta  VariantControl=(inherit)
  Terminator_1 : Terminator
  Terminator_2 : Terminator
  Terminator_3 : Terminator
  u16_DIDNum_LIDAAnchorSta : ArgIn  OutDataTypeStr=uint16  ArgumentName=u16_DIDNum_LIDAAnchorSta
  u16_DIDLen_LIDAAnchorSta : ArgIn  Port=2  OutDataTypeStr=uint16  ArgumentName=u16_DIDLen_LIDAAnchorSta
  u8Array21_LIDAAnchorSta : ArgIn  Port=3  OutDataTypeStr=uint8  PortDimensions=21  ArgumentName=u8Array21_LIDAAnchorSta
  wires:
  u16_DIDNum_LIDAAnchorSta/1 -> Terminator_1/1
  u16_DIDLen_LIDAAnchorSta/1 -> Terminator_2/1
  u8Array21_LIDAAnchorSta/1 -> Terminator_3/1

== system SWC_DID_type/P_DIDWriteCDD/run_DIDSet_LRLowPresThre_sys ==
  function : TriggerPort  TriggerType=function-call  IsSimulinkFunction=on  FunctionName=run_DIDSet_LRLowPresThre  VariantControl=(inherit)
  Terminator_1 : Terminator
  Terminator_2 : Terminator
  Terminator_3 : Terminator
  u16_DIDNum_LRLowPresThre : ArgIn  OutDataTypeStr=uint16  ArgumentName=u16_DIDNum_LRLowPresThre
  u16_DIDLen_LRLowPresThre : ArgIn  Port=2  OutDataTypeStr=uint16  ArgumentName=u16_DIDLen_LRLowPresThre
  u8_LRLowPresThre : ArgIn  Port=3  OutDataTypeStr=uint8  ArgumentName=u8_LRLowPresThre
  wires:
  u16_DIDNum_LRLowPresThre/1 -> Terminator_1/1
  u16_DIDLen_LRLowPresThre/1 -> Terminator_2/1
  u8_LRLowPresThre/1 -> Terminator_3/1

== system SWC_DID_type/P_DIDWriteCDD/run_DIDSet_LRSensorID_sys ==
  function : TriggerPort  TriggerType=function-call  IsSimulinkFunction=on  FunctionName=run_DIDSet_LRSensorID  VariantControl=(inherit)
  Terminator_1 : Terminator
  Terminator_2 : Terminator
  Terminator_3 : Terminator
  u16_DIDNum_LRSensorID : ArgIn  OutDataTypeStr=uint16  ArgumentName=u16_DIDNum_LRSensorID
  u16_DIDLen_LRSensorID : ArgIn  Port=2  OutDataTypeStr=uint16  ArgumentName=u16_DIDLen_LRSensorID
  u8Array4_LRSensorID : ArgIn  Port=3  OutDataTypeStr=uint8  PortDimensions=4  ArgumentName=u8Array4_LRSensorID
  wires:
  u16_DIDNum_LRSensorID/1 -> Terminator_1/1
  u16_DIDLen_LRSensorID/1 -> Terminator_2/1
  u8Array4_LRSensorID/1 -> Terminator_3/1

== system SWC_DID_type/P_DIDWriteCDD/run_DIDSet_MILDIST_sys ==
  note: Added blocks
  note: Added blocks
  note: Added blocks
  note: Added blocks
  function : TriggerPort  TriggerType=function-call  IsSimulinkFunction=on  FunctionName=run_DIDSet_MILDIST  VariantControl=(inherit)
  Terminator_1 : Terminator
  Terminator_2 : Terminator
  Terminator_3 : Terminator
  u16_DIDNum_MILDIST : ArgIn  OutDataTypeStr=uint16  ArgumentName=u16_DIDNum_MILDIST
  u16_DIDLen_MILDIST : ArgIn  Port=2  OutDataTypeStr=uint16  ArgumentName=u16_DIDLen_MILDIST
  u8Array2_MILDIST : ArgIn  Port=3  OutDataTypeStr=uint8  PortDimensions=2  ArgumentName=u8Array2_MILDIST
  wires:
  u16_DIDNum_MILDIST/1 -> Terminator_1/1
  u16_DIDLen_MILDIST/1 -> Terminator_2/1
  u8Array2_MILDIST/1 -> Terminator_3/1

== system SWC_DID_type/P_DIDWriteCDD/run_DIDSet_NUMPSATRIPSFLTMEMCLR_sys ==
  note: Added blocks
  note: Added blocks
  note: Added blocks
  note: Added blocks
  function : TriggerPort  TriggerType=function-call  IsSimulinkFunction=on  FunctionName=run_DIDSet_NUMPSATRIPSFLTMEMCLR  VariantControl=(inherit)
  Terminator_1 : Terminator
  Terminator_2 : Terminator
  Terminator_3 : Terminator
  u16_DIDNum_NUMPSATRIPSFLTMEMCLR : ArgIn  OutDataTypeStr=uint16  ArgumentName=u16_DIDNum_NUMPSATRIPSFLTMEMCLR
  u16_DIDLen_NUMPSATRIPSFLTMEMCLR : ArgIn  Port=2  OutDataTypeStr=uint16  ArgumentName=u16_DIDLen_NUMPSATRIPSFLTMEMCLR
  u8Array2_NUMPSATRIPSFLTMEMCLR : ArgIn  Port=3  OutDataTypeStr=uint8  PortDimensions=2  ArgumentName=u8Array2_NUMPSATRIPSFLTMEMCLR
  wires:
  u16_DIDNum_NUMPSATRIPSFLTMEMCLR/1 -> Terminator_1/1
  u16_DIDLen_NUMPSATRIPSFLTMEMCLR/1 -> Terminator_2/1
  u8Array2_NUMPSATRIPSFLTMEMCLR/1 -> Terminator_3/1

== system SWC_DID_type/P_DIDWriteCDD/run_DIDSet_NVMPedalZP_sys ==
  function : TriggerPort  TriggerType=function-call  IsSimulinkFunction=on  FunctionName=run_DIDSet_NVMPedalZP  VariantControl=(inherit)
  Terminator_1 : Terminator
  Terminator_2 : Terminator
  Terminator_3 : Terminator
  u16_DIDNum_NVMPedalZP : ArgIn  OutDataTypeStr=uint16  ArgumentName=u16_DIDNum_NVMPedalZP
  u16_DIDLen_NVMPedalZP : ArgIn  Port=2  OutDataTypeStr=uint16  ArgumentName=u16_DIDLen_NVMPedalZP
  u8Array3_NVMPedalZP : ArgIn  Port=3  OutDataTypeStr=uint8  PortDimensions=3  ArgumentName=u8Array3_NVMPedalZP
  wires:
  u16_DIDNum_NVMPedalZP/1 -> Terminator_1/1
  u16_DIDLen_NVMPedalZP/1 -> Terminator_2/1
  u8Array3_NVMPedalZP/1 -> Terminator_3/1

== system SWC_DID_type/P_DIDWriteCDD/run_DIDSet_OBDReq_sys ==
  note: Added blocks
  note: Added blocks
  note: Added blocks
  note: Added blocks
  function : TriggerPort  TriggerType=function-call  IsSimulinkFunction=on  FunctionName=run_DIDSet_OBDReq  VariantControl=(inherit)
  Terminator_1 : Terminator
  Terminator_2 : Terminator
  Terminator_3 : Terminator
  u16_DIDNum_OBDReq : ArgIn  OutDataTypeStr=uint16  ArgumentName=u16_DIDNum_OBDReq
  u16_DIDLen_OBDReq : ArgIn  Port=2  OutDataTypeStr=uint16  ArgumentName=u16_DIDLen_OBDReq
  u8_OBDReq : ArgIn  Port=3  OutDataTypeStr=uint8  ArgumentName=u8_OBDReq
  wires:
  u16_DIDNum_OBDReq/1 -> Terminator_1/1
  u16_DIDLen_OBDReq/1 -> Terminator_2/1
  u8_OBDReq/1 -> Terminator_3/1

== system SWC_DID_type/P_DIDWriteCDD/run_DIDSet_ODOMETER_sys ==
  note: Added blocks
  note: Added blocks
  note: Added blocks
  note: Added blocks
  function : TriggerPort  TriggerType=function-call  IsSimulinkFunction=on  FunctionName=run_DIDSet_ODOMETER  VariantControl=(inherit)
  Terminator_1 : Terminator
  Terminator_2 : Terminator
  Terminator_3 : Terminator
  u16_DIDNum_ODOMETER : ArgIn  OutDataTypeStr=uint16  ArgumentName=u16_DIDNum_ODOMETER
  u16_DIDLen_ODOMETER : ArgIn  Port=2  OutDataTypeStr=uint16  ArgumentName=u16_DIDLen_ODOMETER
  u8Array4_ODOMETER : ArgIn  Port=3  OutDataTypeStr=uint8  PortDimensions=4  ArgumentName=u8Array4_ODOMETER
  wires:
  u16_DIDNum_ODOMETER/1 -> Terminator_1/1
  u16_DIDLen_ODOMETER/1 -> Terminator_2/1
  u8Array4_ODOMETER/1 -> Terminator_3/1

== system SWC_DID_type/P_DIDWriteCDD/run_DIDSet_PKE_sys ==
  note: Added blocks
  note: Added blocks
  note: Added blocks
  note: Added blocks
  function : TriggerPort  TriggerType=function-call  IsSimulinkFunction=on  FunctionName=run_DIDSet_PKE  VariantControl=(inherit)
  Terminator_1 : Terminator
  Terminator_2 : Terminator
  Terminator_3 : Terminator
  u16_DIDNum_PKE : ArgIn  OutDataTypeStr=uint16  ArgumentName=u16_DIDNum_PKE
  u16_DIDLen_PKE : ArgIn  Port=2  OutDataTypeStr=uint16  ArgumentName=u16_DIDLen_PKE
  u8Array8_PKE : ArgIn  Port=3  OutDataTypeStr=uint8  PortDimensions=8  ArgumentName=u8Array8_PKE
  wires:
  u16_DIDNum_PKE/1 -> Terminator_1/1
  u16_DIDLen_PKE/1 -> Terminator_2/1
  u8Array8_PKE/1 -> Terminator_3/1

== system SWC_DID_type/P_DIDWriteCDD/run_DIDSet_PSA_sys ==
  note: Added blocks
  note: Added blocks
  note: Added blocks
  note: Added blocks
  function : TriggerPort  TriggerType=function-call  IsSimulinkFunction=on  FunctionName=run_DIDSet_PSA  VariantControl=(inherit)
  Terminator_1 : Terminator
  Terminator_2 : Terminator
  Terminator_3 : Terminator
  u16_DIDNum_PSA : ArgIn  OutDataTypeStr=uint16  ArgumentName=u16_DIDNum_PSA
  u16_DIDLen_PSA : ArgIn  Port=2  OutDataTypeStr=uint16  ArgumentName=u16_DIDLen_PSA
  u8Array24_PSA : ArgIn  Port=3  OutDataTypeStr=uint8  PortDimensions=24  ArgumentName=u8Array24_PSA
  wires:
  u16_DIDNum_PSA/1 -> Terminator_1/1
  u16_DIDLen_PSA/1 -> Terminator_2/1
  u8Array24_PSA/1 -> Terminator_3/1

== system SWC_DID_type/P_DIDWriteCDD/run_DIDSet_ProtocolId_sys ==
  note: Added blocks
  note: Added blocks
  note: Added blocks
  note: Added blocks
  function : TriggerPort  TriggerType=function-call  IsSimulinkFunction=on  FunctionName=run_DIDSet_ProtocolId  VariantControl=(inherit)
  Terminator_1 : Terminator
  Terminator_2 : Terminator
  Terminator_3 : Terminator
  u16_DIDNum_ProtocolId : ArgIn  OutDataTypeStr=uint16  ArgumentName=u16_DIDNum_ProtocolId
  u16_DIDLen_ProtocolId : ArgIn  Port=2  OutDataTypeStr=uint16  ArgumentName=u16_DIDLen_ProtocolId
  u8_ProtocolId : ArgIn  Port=3  OutDataTypeStr=uint8  ArgumentName=u8_ProtocolId
  wires:
  u16_DIDNum_ProtocolId/1 -> Terminator_1/1
  u16_DIDLen_ProtocolId/1 -> Terminator_2/1
  u8_ProtocolId/1 -> Terminator_3/1

== system SWC_DID_type/P_DIDWriteCDD/run_DIDSet_QTYPSATRIPS_sys ==
  note: Added blocks
  note: Added blocks
  note: Added blocks
  note: Added blocks
  function : TriggerPort  TriggerType=function-call  IsSimulinkFunction=on  FunctionName=run_DIDSet_QTYPSATRIPS  VariantControl=(inherit)
  Terminator_1 : Terminator
  Terminator_2 : Terminator
  Terminator_3 : Terminator
  u16_DIDNum_QTYPSATRIPS : ArgIn  OutDataTypeStr=uint16  ArgumentName=u16_DIDNum_QTYPSATRIPS
  u16_DIDLen_QTYPSATRIPS : ArgIn  Port=2  OutDataTypeStr=uint16  ArgumentName=u16_DIDLen_QTYPSATRIPS
  u8Array8_QTYPSATRIPS : ArgIn  Port=3  OutDataTypeStr=uint8  PortDimensions=8  ArgumentName=u8Array8_QTYPSATRIPS
  wires:
  u16_DIDNum_QTYPSATRIPS/1 -> Terminator_1/1
  u16_DIDLen_QTYPSATRIPS/1 -> Terminator_2/1
  u8Array8_QTYPSATRIPS/1 -> Terminator_3/1

== system SWC_DID_type/P_DIDWriteCDD/run_DIDSet_RFLowPresThre_sys ==
  function : TriggerPort  TriggerType=function-call  IsSimulinkFunction=on  FunctionName=run_DIDSet_RFLowPresThre  VariantControl=(inherit)
  Terminator_1 : Terminator
  Terminator_2 : Terminator
  Terminator_3 : Terminator
  u16_DIDNum_RFLowPresThre : ArgIn  OutDataTypeStr=uint16  ArgumentName=u16_DIDNum_RFLowPresThre
  u16_DIDLen_RFLowPresThre : ArgIn  Port=2  OutDataTypeStr=uint16  ArgumentName=u16_DIDLen_RFLowPresThre
  u8_RFLowPresThre : ArgIn  Port=3  OutDataTypeStr=uint8  ArgumentName=u8_RFLowPresThre
  wires:
  u16_DIDNum_RFLowPresThre/1 -> Terminator_1/1
  u16_DIDLen_RFLowPresThre/1 -> Terminator_2/1
  u8_RFLowPresThre/1 -> Terminator_3/1

== system SWC_DID_type/P_DIDWriteCDD/run_DIDSet_RFSensorID_sys ==
  function : TriggerPort  TriggerType=function-call  IsSimulinkFunction=on  FunctionName=run_DIDSet_RFSensorID  VariantControl=(inherit)
  Terminator_1 : Terminator
  Terminator_2 : Terminator
  Terminator_3 : Terminator
  u16_DIDNum_RFSensorID : ArgIn  OutDataTypeStr=uint16  ArgumentName=u16_DIDNum_RFSensorID
  u16_DIDLen_RFSensorID : ArgIn  Port=2  OutDataTypeStr=uint16  ArgumentName=u16_DIDLen_RFSensorID
  u8Array4_RFSensorID : ArgIn  Port=3  OutDataTypeStr=uint8  PortDimensions=4  ArgumentName=u8Array4_RFSensorID
  wires:
  u16_DIDNum_RFSensorID/1 -> Terminator_1/1
  u16_DIDLen_RFSensorID/1 -> Terminator_2/1
  u8Array4_RFSensorID/1 -> Terminator_3/1

== system SWC_DID_type/P_DIDWriteCDD/run_DIDSet_RRLowPresThre_sys ==
  function : TriggerPort  TriggerType=function-call  IsSimulinkFunction=on  FunctionName=run_DIDSet_RRLowPresThre  VariantControl=(inherit)
  Terminator_1 : Terminator
  Terminator_2 : Terminator
  Terminator_3 : Terminator
  u16_DIDNum_RRLowPresThre : ArgIn  OutDataTypeStr=uint16  ArgumentName=u16_DIDNum_RRLowPresThre
  u16_DIDLen_RRLowPresThre : ArgIn  Port=2  OutDataTypeStr=uint16  ArgumentName=u16_DIDLen_RRLowPresThre
  u8_RRLowPresThre : ArgIn  Port=3  OutDataTypeStr=uint8  ArgumentName=u8_RRLowPresThre
  wires:
  u16_DIDNum_RRLowPresThre/1 -> Terminator_1/1
  u16_DIDLen_RRLowPresThre/1 -> Terminator_2/1
  u8_RRLowPresThre/1 -> Terminator_3/1

== system SWC_DID_type/P_DIDWriteCDD/run_DIDSet_RRSensorID_sys ==
  function : TriggerPort  TriggerType=function-call  IsSimulinkFunction=on  FunctionName=run_DIDSet_RRSensorID  VariantControl=(inherit)
  Terminator_1 : Terminator
  Terminator_2 : Terminator
  Terminator_3 : Terminator
  u16_DIDNum_RRSensorID : ArgIn  OutDataTypeStr=uint16  ArgumentName=u16_DIDNum_RRSensorID
  u16_DIDLen_RRSensorID : ArgIn  Port=2  OutDataTypeStr=uint16  ArgumentName=u16_DIDLen_RRSensorID
  u8Array4_RRSensorID : ArgIn  Port=3  OutDataTypeStr=uint8  PortDimensions=4  ArgumentName=u8Array4_RRSensorID
  wires:
  u16_DIDNum_RRSensorID/1 -> Terminator_1/1
  u16_DIDLen_RRSensorID/1 -> Terminator_2/1
  u8Array4_RRSensorID/1 -> Terminator_3/1
